simulink model "sender"  (R2021b)
settings: Solver=VariableStepAuto  StartTime=0.0  StopTime=inf  RelTol=1e-3
settings Model: Creator=VVasco  LastModifiedBy=vgaggero

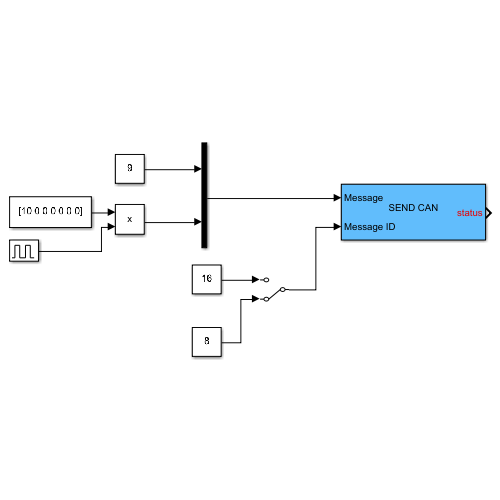
[thumbnail: Simulink's stored preview of the top-level diagram]
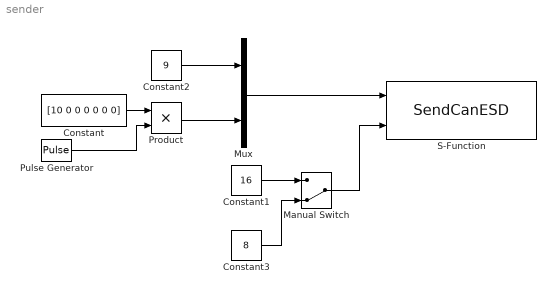
== system sender ==
  Constant : Constant  Value=[10 0 0 0 0 0 0]
  Constant1 : Constant  Value=16
  Constant2 : Constant  Value=9
  Constant3 : Constant  Value=8
  Manual Switch : ManualSwitch  CurrentSetting=0
  Mux : Mux  Inputs=2
  Product : Product
  Pulse Generator : DiscretePulseGenerator  PulseType=Time based  Period=0.5  PulseWidth=50
  S-Function : S-Function  FunctionName=SendCanESD  Parameters=(baudrate-1),netid,length, txQueueSize, rxQueueSize, txTimeout, rxTimeout  SFunctionDeploymentMode=off  EnableBusSupport=off  mask{baudrate=1000 Kbit/s, netid=0, length=8, txQueueSize=1, rxQueueSize=1, txTimeout=0, rxTimeout=0}
      mask prompts: netid "CAN Network"; length "Message Length"; txQueueSize "Tx queue size"; rxQueueSize "Rx queue size"; txTimeout "Tx timeout"; rxTimeout "Rx timeout"
      mask TypeOptions baudrate: 1000 Kbit/s | 500 Kbit/s
      mask Display:
      | fprintf('SEND CAN\n')
      | port_label('input',1,'Message');
      | port_label('input',2,'Message ID');
      | color('red');port_label('output',1,'status');
  wires:
  Pulse Generator/1 -> Product/2
  Constant/1 -> Product/1
  Mux/1 -> S-Function/1
  Product/1 -> Mux/2
  Constant2/1 -> Mux/1
  Constant1/1 -> Manual Switch/1
  Constant3/1 -> Manual Switch/2
  Manual Switch/1 -> S-Function/2
